simulink model "silnikDC_bezwladnosc"  (R2017b)
settings: Solver=ode3  StartTime=0.0  StopTime=100  FixedStep=100e-6  MaxStep=0.0001  RelTol=1e-3  EnableMultiTasking=on
InitFcn:
  | parametryDC;
values from neighbouring files (symbols this model uses):
  a = 0.7    [parametryDC.m]
  B = 0.002953    [parametryDC.m]
  J = 0.02215    [parametryDC.m]
  K = 1.28    [parametryDC.m]
  k1 = 1.28    [parametryDC.m]
  La = 0.1215    [parametryDC.m]
  Ra = 11.2    [parametryDC.m]
libraries: simulink x3
settings Model: Creator=Siembab  LastModifiedBy=AW
settings SolverCC: ZeroCrossAlgorithm=Adaptive
settings DataIOCC: LimitDataPoints=on  SaveFormat=Array  SignalLoggingSaveFormat=ModelDataLogs
settings OptimizationCC: ExpressionDepthLimit=2147483647  LifeSpan=inf
settings DebuggingCC: UnderspecifiedInitializationDetection=Classic  MergeDetectMultiDrivingBlocksExec=none  SolverPrmCheckMsg=warning  FcnCallInpInsideContextMsg=warning  StateNameClashWarn=warning  SFUnexpectedBacktrackingDiag=warning  SFNoUnconditionalDefaultTransitionDiag=warning  SFExecutionAtInitializationDiag=none
settings HardwareCC: ProdBitPerPointer=32  ProdBitPerSizeT=32  ProdBitPerPtrDiffT=32  ProdLargestAtomicFloat=None  ProdIntDivRoundTo=Undefined  ProdEndianess=Unspecified  ProdWordSize=32  ProdHWDeviceType=32-bit Generic
settings ModelReferenceCC: PropagateSignalLabelsOutOfModel=off
settings CodeAppCC: StateflowObjectComments=on
settings GRTTargetCC: TargetLangStandard=C89/C90 (ANSI)  GeneratePreprocessorConditionals=Disable all  CombineOutputUpdateFcns=off  GRTInterface=on
settings ConfigComp: CovMetricSettings=dw  CovHtmlReporting=on  CovSaveCumulativeToWorkspaceVar=on  CovSaveSingleToWorkspaceVar=on  CovExternalEMLEnable=off

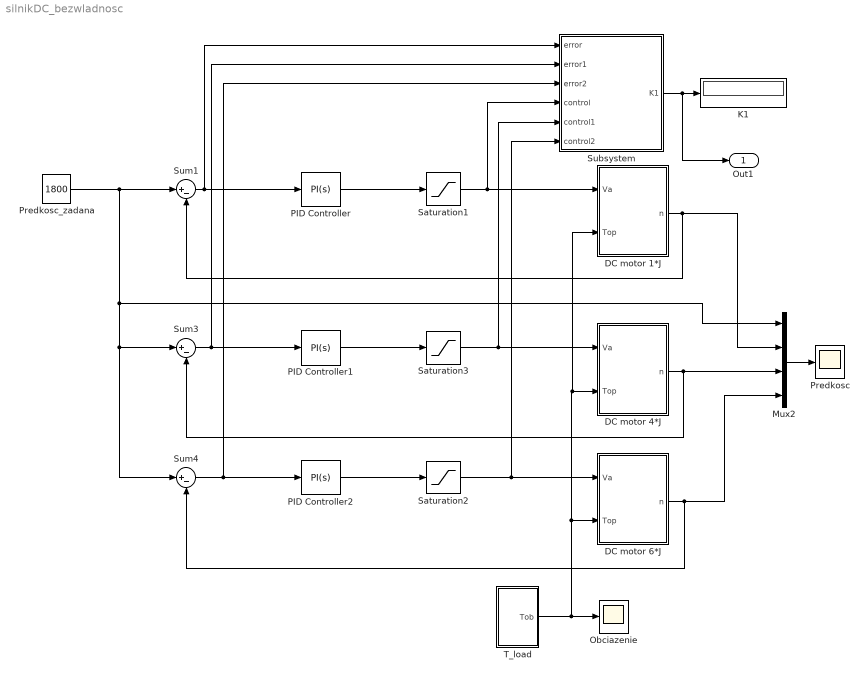
== system silnikDC_bezwladnosc ==
  DC motor 1*J : Subsystem
  DC motor 4*J : Subsystem
  DC motor 6*J : Subsystem
  K1 : Display
  Mux2 : Mux
  Obciazenie : Scope
  PID Controller : simulink/Continuous/PID Controller  Controller=PI  TimeDomain=Continuous-time  SampleTime=-1  IntegratorMethod=Forward Euler  FilterMethod=Forward Euler  Form=Parallel  UseFilter=on  ControllerParametersSource=internal  P=1.0116  I=4.2829  D=0.000552703256129822  N=198.815285878902  InitialConditionSource=internal  InitialConditionForIntegrator=0  InitialConditionForFilter=0  ExternalReset=none  LimitOutput=off  UpperSaturationLimit=inf  LowerSaturationLimit=-inf  LinearizeAsGain=off  AntiWindupMode=none  Kb=1  TrackingMode=off  Kt=1  PParamMin=[]  PParamMax=[]  IParamMin=[]  IParamMax=[]  DParamMin=[]  DParamMax=[]  NParamMin=[]  NParamMax=[]  KbParamMin=[]  KbParamMax=[]  KtParamMin=[]  KtParamMax=[]  POutMin=[]  POutMax=[]  IOutMin=[]  IOutMax=[]  DOutMin=[]  DOutMax=[]  NOutMin=[]  NOutMax=[]  KbOutMin=[]  KbOutMax=[]  KtOutMin=[]  KtOutMax=[]  IntegratorOutMin=[]  IntegratorOutMax=[]  FilterOutMin=[]  FilterOutMax=[]  SumOutMin=[]  SumOutMax=[]  SumI1OutMin=[]  SumI1OutMax=[]  SumI2OutMin=[]  SumI2OutMax=[]  SumI3OutMin=[]  SumI3OutMax=[]  SumDOutMin=[]  SumDOutMax=[]  SaturationOutMin=[]  SaturationOutMax=[]  IntegratorContinuousStateAttributes=''  IntegratorStateMustResolveToSignalObject=off  IntegratorRTWStateStorageClass=Auto  FilterContinuousStateAttributes=''  FilterStateMustResolveToSignalObject=off  FilterRTWStateStorageClass=Auto  DifferentiatorICPrevScaledInput=0  DifferentiatorOutMin=[]  DifferentiatorOutMax=[]  InitialConditionSetting=State (most efficient)  FilterDiffOutCoefMin=[]  FilterDiffOutCoefMax=[]  SumDenOutMin=[]  SumDenOutMax=[]  SumNumOutMin=[]  SumNumOutMax=[]  ReciprocalOutMin=[]  ReciprocalOutMax=[]  DivideOutMin=[]  DivideOutMax=[]  TunerSelectOption=Transfer Function Based (PID Tuner App)
  PID Controller1 : simulink/Continuous/PID Controller  Controller=PI  TimeDomain=Continuous-time  SampleTime=-1  IntegratorMethod=Forward Euler  FilterMethod=Forward Euler  Form=Parallel  UseFilter=on  ControllerParametersSource=internal  P=0.64519  I=2.2953  D=0.000552703256129822  N=198.815285878902  InitialConditionSource=internal  InitialConditionForIntegrator=0  InitialConditionForFilter=0  ExternalReset=none  LimitOutput=off  UpperSaturationLimit=inf  LowerSaturationLimit=-inf  LinearizeAsGain=off  AntiWindupMode=none  Kb=1  TrackingMode=off  Kt=1  PParamMin=[]  PParamMax=[]  IParamMin=[]  IParamMax=[]  DParamMin=[]  DParamMax=[]  NParamMin=[]  NParamMax=[]  KbParamMin=[]  KbParamMax=[]  KtParamMin=[]  KtParamMax=[]  POutMin=[]  POutMax=[]  IOutMin=[]  IOutMax=[]  DOutMin=[]  DOutMax=[]  NOutMin=[]  NOutMax=[]  KbOutMin=[]  KbOutMax=[]  KtOutMin=[]  KtOutMax=[]  IntegratorOutMin=[]  IntegratorOutMax=[]  FilterOutMin=[]  FilterOutMax=[]  SumOutMin=[]  SumOutMax=[]  SumI1OutMin=[]  SumI1OutMax=[]  SumI2OutMin=[]  SumI2OutMax=[]  SumI3OutMin=[]  SumI3OutMax=[]  SumDOutMin=[]  SumDOutMax=[]  SaturationOutMin=[]  SaturationOutMax=[]  IntegratorContinuousStateAttributes=''  IntegratorStateMustResolveToSignalObject=off  IntegratorRTWStateStorageClass=Auto  FilterContinuousStateAttributes=''  FilterStateMustResolveToSignalObject=off  FilterRTWStateStorageClass=Auto  DifferentiatorICPrevScaledInput=0  DifferentiatorOutMin=[]  DifferentiatorOutMax=[]  InitialConditionSetting=State (most efficient)  FilterDiffOutCoefMin=[]  FilterDiffOutCoefMax=[]  SumDenOutMin=[]  SumDenOutMax=[]  SumNumOutMin=[]  SumNumOutMax=[]  ReciprocalOutMin=[]  ReciprocalOutMax=[]  DivideOutMin=[]  DivideOutMax=[]  TunerSelectOption=Transfer Function Based (PID Tuner App)
  PID Controller2 : simulink/Continuous/PID Controller  Controller=PI  TimeDomain=Continuous-time  SampleTime=-1  IntegratorMethod=Forward Euler  FilterMethod=Forward Euler  Form=Parallel  UseFilter=on  ControllerParametersSource=internal  P=0.87064  I=1.5675  D=0.000552703256129822  N=198.815285878902  InitialConditionSource=internal  InitialConditionForIntegrator=0  InitialConditionForFilter=0  ExternalReset=none  LimitOutput=off  UpperSaturationLimit=inf  LowerSaturationLimit=-inf  LinearizeAsGain=off  AntiWindupMode=none  Kb=1  TrackingMode=off  Kt=1  PParamMin=[]  PParamMax=[]  IParamMin=[]  IParamMax=[]  DParamMin=[]  DParamMax=[]  NParamMin=[]  NParamMax=[]  KbParamMin=[]  KbParamMax=[]  KtParamMin=[]  KtParamMax=[]  POutMin=[]  POutMax=[]  IOutMin=[]  IOutMax=[]  DOutMin=[]  DOutMax=[]  NOutMin=[]  NOutMax=[]  KbOutMin=[]  KbOutMax=[]  KtOutMin=[]  KtOutMax=[]  IntegratorOutMin=[]  IntegratorOutMax=[]  FilterOutMin=[]  FilterOutMax=[]  SumOutMin=[]  SumOutMax=[]  SumI1OutMin=[]  SumI1OutMax=[]  SumI2OutMin=[]  SumI2OutMax=[]  SumI3OutMin=[]  SumI3OutMax=[]  SumDOutMin=[]  SumDOutMax=[]  SaturationOutMin=[]  SaturationOutMax=[]  IntegratorContinuousStateAttributes=''  IntegratorStateMustResolveToSignalObject=off  IntegratorRTWStateStorageClass=Auto  FilterContinuousStateAttributes=''  FilterStateMustResolveToSignalObject=off  FilterRTWStateStorageClass=Auto  DifferentiatorICPrevScaledInput=0  DifferentiatorOutMin=[]  DifferentiatorOutMax=[]  InitialConditionSetting=State (most efficient)  FilterDiffOutCoefMin=[]  FilterDiffOutCoefMax=[]  SumDenOutMin=[]  SumDenOutMax=[]  SumNumOutMin=[]  SumNumOutMax=[]  ReciprocalOutMin=[]  ReciprocalOutMax=[]  DivideOutMin=[]  DivideOutMax=[]  TunerSelectOption=Transfer Function Based (PID Tuner App)
  Predkosc : Scope
  Predkosc_zadana : Constant  Value=1800
  Saturation1 : Saturate  UpperLimit=500  LowerLimit=-500
  Saturation2 : Saturate  UpperLimit=500  LowerLimit=-500
  Saturation3 : Saturate  UpperLimit=500  LowerLimit=-500
  Subsystem : Subsystem
  Sum1 : Sum  Inputs=|+-
  Sum3 : Sum  Inputs=|+-
  Sum4 : Sum  Inputs=|+-
  T_load : Subsystem
  Out1 : Outport
  wires:
  Saturation1/1 -> Subsystem/4(control), DC motor 1*J/1(Va)
  Predkosc_zadana/1 -> Mux2/1, Sum4/1, Sum3/1, Sum1/1
  DC motor 1*J/1(n) -> Mux2/2, Sum1/2
  Mux2/1 -> Predkosc/1
  DC motor 6*J/1(n) -> Sum4/2, Mux2/4
  DC motor 4*J/1(n) -> Sum3/2, Mux2/3
  PID Controller2/1 -> Saturation2/1
  Saturation2/1 -> Subsystem/6(control2), DC motor 6*J/1(Va)
  PID Controller1/1 -> Saturation3/1
  Saturation3/1 -> Subsystem/5(control1), DC motor 4*J/1(Va)
  Sum3/1 -> Subsystem/2(error1), PID Controller1/1
  Sum4/1 -> Subsystem/3(error2), PID Controller2/1
  PID Controller/1 -> Saturation1/1
  Sum1/1 -> Subsystem/1(error), PID Controller/1
  T_load/1(Tob) -> Obciazenie/1, DC motor 1*J/2(Top), DC motor 4*J/2(Top), DC motor 6*J/2(Top)
  Subsystem/1(K1) -> Out1/1, K1/1

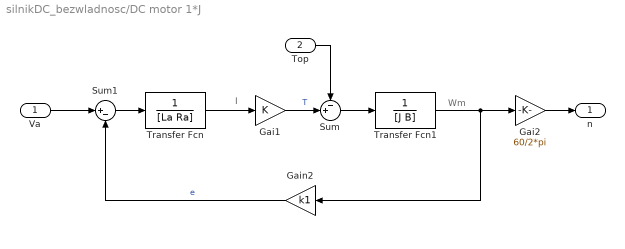
== system silnikDC_bezwladnosc/DC motor 1*J ==
  note: Wm
  note: I
  Va : Inport
  Top : Inport  Port=2
  Gai1 : Gain  Gain=K
  Gai2 : Gain  Gain=60/2*pi
  Gain2 : Gain  Gain=k1
  Sum : Sum  Inputs=-+|
  Sum1 : Sum  Inputs=|+-
  Transfer Fcn : TransferFcn  Denominator=[La Ra]
  Transfer Fcn1 : TransferFcn  Denominator=[J B]
  n : Outport
  wires:
  Transfer Fcn/1 -> Gai1/1
  Gai1/1 -> Sum/2  "T"
  Sum/1 -> Transfer Fcn1/1
  Gain2/1 -> Sum1/2  "e"
  Transfer Fcn1/1 -> Gai2/1, Gain2/1
  Sum1/1 -> Transfer Fcn/1
  Va/1 -> Sum1/1
  Top/1 -> Sum/1
  Gai2/1 -> n/1

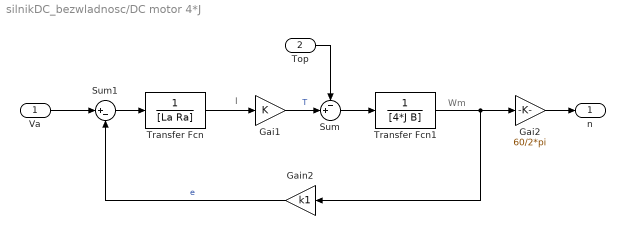
== system silnikDC_bezwladnosc/DC motor 4*J ==
  note: Wm
  note: I
  Va : Inport
  Top : Inport  Port=2
  Gai1 : Gain  Gain=K
  Gai2 : Gain  Gain=60/2*pi
  Gain2 : Gain  Gain=k1
  Sum : Sum  Inputs=-+|
  Sum1 : Sum  Inputs=|+-
  Transfer Fcn : TransferFcn  Denominator=[La Ra]
  Transfer Fcn1 : TransferFcn  Denominator=[4*J B]
  n : Outport
  wires:
  Transfer Fcn/1 -> Gai1/1
  Gai1/1 -> Sum/2  "T"
  Sum/1 -> Transfer Fcn1/1
  Gain2/1 -> Sum1/2  "e"
  Transfer Fcn1/1 -> Gai2/1, Gain2/1
  Sum1/1 -> Transfer Fcn/1
  Va/1 -> Sum1/1
  Top/1 -> Sum/1
  Gai2/1 -> n/1

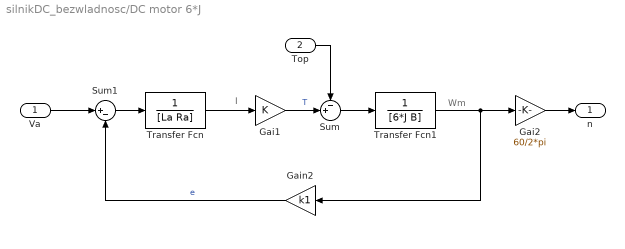
== system silnikDC_bezwladnosc/DC motor 6*J ==
  note: Wm
  note: I
  Va : Inport
  Top : Inport  Port=2
  Gai1 : Gain  Gain=K
  Gai2 : Gain  Gain=60/2*pi
  Gain2 : Gain  Gain=k1
  Sum : Sum  Inputs=-+|
  Sum1 : Sum  Inputs=|+-
  Transfer Fcn : TransferFcn  Denominator=[La Ra]
  Transfer Fcn1 : TransferFcn  Denominator=[6*J B]
  n : Outport
  wires:
  Transfer Fcn/1 -> Gai1/1
  Gai1/1 -> Sum/2  "T"
  Sum/1 -> Transfer Fcn1/1
  Gain2/1 -> Sum1/2  "e"
  Transfer Fcn1/1 -> Gai2/1, Gain2/1
  Sum1/1 -> Transfer Fcn/1
  Va/1 -> Sum1/1
  Top/1 -> Sum/1
  Gai2/1 -> n/1

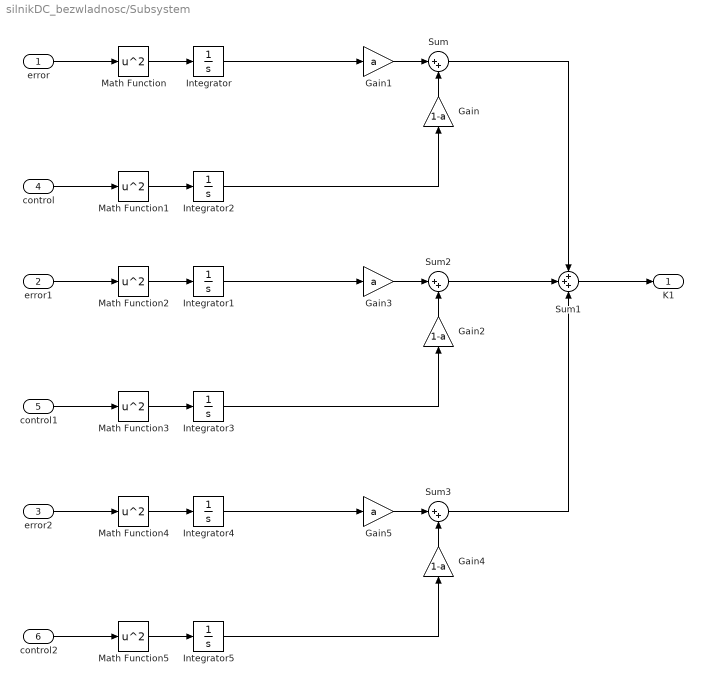
== system silnikDC_bezwladnosc/Subsystem ==
  error : Inport
  error1 : Inport  Port=2
  error2 : Inport  Port=3
  control : Inport  Port=4
  control1 : Inport  Port=5
  control2 : Inport  Port=6
  Gain : Gain  Gain=1-a
  Gain1 : Gain  Gain=a
  Gain2 : Gain  Gain=1-a
  Gain3 : Gain  Gain=a
  Gain4 : Gain  Gain=1-a
  Gain5 : Gain  Gain=a
  Integrator{,1..5} (6 alike) : Integrator
  Math Function{,1..5} (6 alike) : Math  Operator=square  SaturateOnIntegerOverflow=on
  Sum : Sum  Inputs=|++
  Sum1 : Sum  Inputs=+++
  Sum2 : Sum  Inputs=|++
  Sum3 : Sum  Inputs=|++
  K1 : Outport
  wires:
  Integrator2/1 -> Gain/1
  Math Function1/1 -> Integrator2/1
  Gain/1 -> Sum/2
  Gain1/1 -> Sum/1
  Math Function/1 -> Integrator/1
  Integrator/1 -> Gain1/1
  error/1 -> Math Function/1
  control/1 -> Math Function1/1
  Integrator3/1 -> Gain2/1
  Math Function3/1 -> Integrator3/1
  Gain2/1 -> Sum2/2
  Gain3/1 -> Sum2/1
  Math Function2/1 -> Integrator1/1
  Integrator1/1 -> Gain3/1
  error1/1 -> Math Function2/1
  control1/1 -> Math Function3/1
  Integrator5/1 -> Gain4/1
  Math Function5/1 -> Integrator5/1
  Gain4/1 -> Sum3/2
  Gain5/1 -> Sum3/1
  Math Function4/1 -> Integrator4/1
  Integrator4/1 -> Gain5/1
  error2/1 -> Math Function4/1
  control2/1 -> Math Function5/1
  Sum2/1 -> Sum1/2
  Sum3/1 -> Sum1/3
  Sum/1 -> Sum1/1
  Sum1/1 -> K1/1

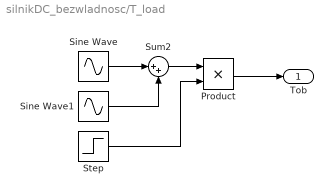
== system silnikDC_bezwladnosc/T_load ==
  Product : Product
  Sine Wave : Sin  Amplitude=8  Bias=10  Frequency=100  SampleTime=0
  Sine Wave1 : Sin  Amplitude=8/3  Bias=10  Frequency=3*100  SampleTime=0
  Step : Step  Time=0.5  SampleTime=0
  Sum2 : Sum  Inputs=|++
  Tob : Outport
  wires:
  Sum2/1 -> Product/1
  Sine Wave1/1 -> Sum2/2
  Sine Wave/1 -> Sum2/1
  Step/1 -> Product/2
  Product/1 -> Tob/1
